simulink model "sampleModel1932"  (R2023a)
settings: Solver=VariableStepAuto  StartTime=0.0  StopTime=10.0  RelTol=1e-3
libraries: hdlsllib x4, simulink x3
settings Model: Creator=user1  LastModifiedBy=user1

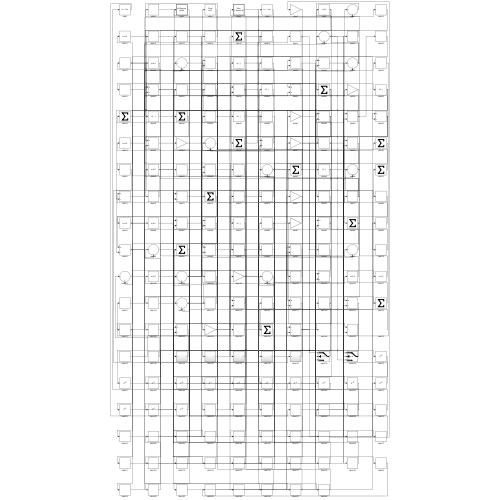
[thumbnail: Simulink's stored preview of the top-level diagram]
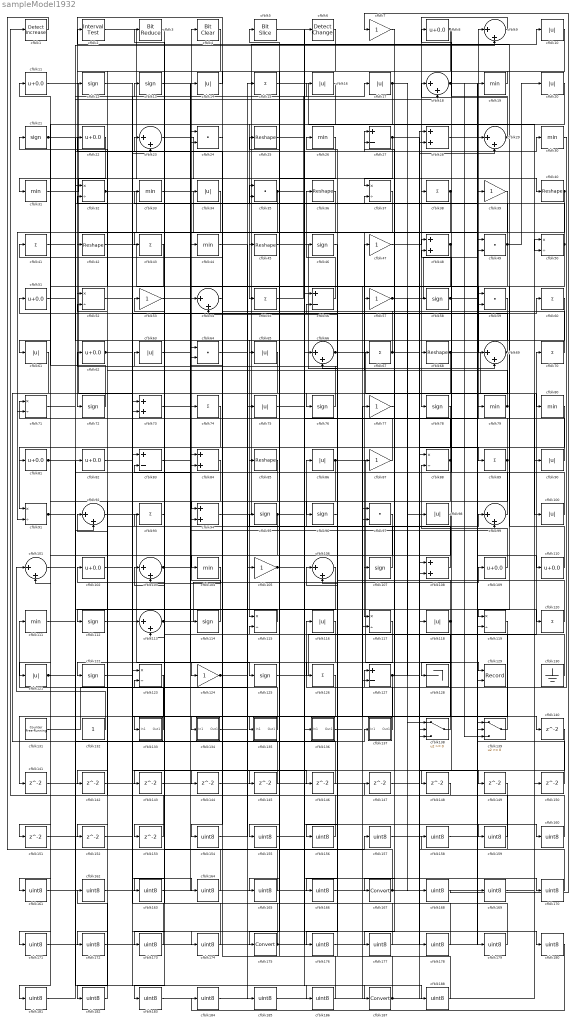
== system sampleModel1932 ==
  cfblk1 : simulink/Logic and Bit Operations/Detect Increase  vinit=0.0  OutDataTypeStr=boolean
      settings: LibrarySourceBlock=|
      | hdlsllib/Logic and Bit
      | Operations/Detect
      | Increase
  cfblk{10,14,16..17,20,34,61,63,65,75,86,90,98,100,116,118,121} (17 alike) : Abs  SaturateOnIntegerOverflow=off
  cfblk{9,18,23,29,54,66,69,92,99,101,103,106,113} (13 alike) : Sum  Inputs=|++
  cfblk{8,11,22,51,62,81..82,102,109..110} (10 alike) : Bias  Bias=0.0  SaturateOnIntegerOverflow=off
  cfblk{19,26,30..31,33,44,79..80,104,111} (10 alike) : MinMax
  cfblk{7,39,47,53,57,77,87,105,124} (9 alike) : Gain
  cfblk{12..13,21,46,58,72,76,78,95..96,107,112,114,122,125} (15 alike) : Signum
  cfblk{28,48,73,84,94,108} (6 alike) : Sum
  cfblk{32,37,50,52,71,88,91,115,117,119,123} (11 alike) : Product  Inputs=*/  RndMeth=Zero  SaturateOnIntegerOverflow=on
  cfblk{15,38,41,43,55,60,67,70,74,89,93,120,126} (13 alike) : Sum  Inputs=+
  cfblk{27,56,83,127} (4 alike) : Sum  Inputs=+-
  cfblk128 : Terminator
  cfblk129 : Record  FileSettingsInternal="{\"entries\":[{\"content\":{\"excelSettings\":{\"content\":{},\"type\":\"Streamout.ExcelSettings\"}},\"type\":\"Streamout.FileSettingStorage\",\"uuid\":\"\"}],\"packageUris\":[\"http:\\/\\/schema.mathworks.com\\/mf0\\/streamout_blocks\\/R2020a\"],\"version\":\"1.0\"}"  Layout=[1 1]  SignalsInternal="{\"entries\":[{\"content\":{\"signals\":[{\"content\":{\"blockPath\":[],\"dimensions\":[1],\"domain\":\"\",\"lineColor\":\"#a2142f\",\"plots\":[1],\"port\":1,\"signalID\":5289,\"signalName\":\"XY Graph:1\"},\"type\":\"RecordBlkView.Signal\",\"uuid\":\"\"},{\"content\":{\"blockPath\":[],\"dimensions\":[1],\"domain\":\"\",\"lineColor\":\"#139fff\",\"plots\":[1],\"port\":2,\"signalID\":5292,\"signalName\":\"XY Graph:2\"},\"type\":\"RecordBlkView.Signal\",\"uuid\":\"\"}]},\"type\":\"RecordBlkView.InputSignals\",\"uuid\":\"\"}],\"packageUris\":[\"http:\\/\\/schema.mathworks.com\\/mf0\\/streamout_blocks\\/R2020a\"],\"version\":\"1.0\"}"  VisualizationBindings="{\"xyplotplugin\":{\"info\":[{\"series\":[{\"bindingParametersList\":[{\"parameter\":\"X-Axis\",\"signalID\":5289,\"signalName\":\"XY Graph:1\"},{\"parameter\":\"Y-Axis\",\"signalID\":5292,\"signalName\":\"XY Graph:2\"}],\"seriesID\":37715}],\"subplotID\":1}]}}"  CompatibilityTag=XY  st=-1
  cfblk130 : Ground
  cfblk131 : hdlsllib/Sources/Counter Free-Running  NumBits=16  tsamp=-1
  cfblk132 : Constant  SampleTime=-1
  cfblk133 : Subsystem
      settings: LibrarySourceBlock=|
      | hdlsllib/Ports &
      | Subsystems/Subsystem
  cfblk134 : Subsystem
      settings: LibrarySourceBlock=|
      | hdlsllib/Ports &
      | Subsystems/Subsystem
  cfblk135 : Subsystem
      settings: LibrarySourceBlock=|
      | hdlsllib/Ports &
      | Subsystems/Subsystem
  cfblk136 : Subsystem
      settings: LibrarySourceBlock=|
      | hdlsllib/Ports &
      | Subsystems/Subsystem
  cfblk137 : Subsystem
      settings: LibrarySourceBlock=|
      | hdlsllib/Ports &
      | Subsystems/Subsystem
  cfblk138 : Switch  SaturateOnIntegerOverflow=off  InputSameDT=off
  cfblk139 : Switch  SaturateOnIntegerOverflow=off  InputSameDT=off
  cfblk{140..153} (14 alike) : Delay  SampleTime=1
  cfblk{154..166,168..174,176..186,188} (32 alike) : DataTypeConversion  OutDataTypeStr=uint8  SaturateOnIntegerOverflow=off  RndMeth=Floor
  cfblk167 : DataTypeConversion  SaturateOnIntegerOverflow=off  RndMeth=Floor
  cfblk175 : DataTypeConversion  SaturateOnIntegerOverflow=off  RndMeth=Floor
  cfblk187 : DataTypeConversion  SaturateOnIntegerOverflow=off  RndMeth=Floor
  cfblk2 : hdlsllib/Logic and Bit Operations/Interval Test  IntervalClosedRight=on  uplimit=0.5  IntervalClosedLeft=on  lowlimit=-0.5  OutDataTypeStr=boolean
  cfblk{24,35,49,59,64,97} (6 alike) : DotProduct  OutDataTypeStr=Inherit: Inherit via internal rule
  cfblk{25,36,40,42,45,68,85} (7 alike) : Reshape
  cfblk3 : hdlsllib/Logic and Bit Operations/Bit Reduce  mode=AND
  cfblk4 : simulink/Logic and Bit Operations/Bit Clear  iBit=0
      settings: LibrarySourceBlock=|
      | hdlsllib/Logic and Bit
      | Operations/Bit Clear
  cfblk5 : hdlsllib/Logic and Bit Operations/Bit Slice  lidx=7  ridx=0
  cfblk6 : simulink/Logic and Bit Operations/Detect Change  vinit=0  OutDataTypeStr=boolean
      settings: LibrarySourceBlock=|
      | hdlsllib/Logic and Bit
      | Operations/Detect
      | Change
  wires:
  cfblk86/1 -> cfblk129/1, cfblk113/2
  cfblk114/1 -> cfblk4/1
  cfblk133/1(Out1) -> cfblk111/1
  cfblk92/1 -> cfblk124/1
  cfblk90/1 -> cfblk9/1
  cfblk78/1 -> cfblk91/1
  cfblk14/1 -> cfblk72/1
  cfblk56/1 -> cfblk36/1
  cfblk55/1 -> cfblk17/1
  cfblk9/1 -> cfblk78/1
  cfblk49/1 -> cfblk25/1, cfblk20/1, cfblk166/1
  cfblk30/1 -> cfblk116/1
  cfblk107/1 -> cfblk21/1
  cfblk113/1 -> cfblk109/1, cfblk125/1
  cfblk137/1(Out1) -> cfblk127/1
  cfblk126/1 -> cfblk133/1(In1)
  cfblk115/1 -> cfblk112/1
  cfblk63/1 -> cfblk60/1
  cfblk37/1 -> cfblk117/1
  cfblk60/1 -> cfblk115/1
  cfblk118/1 -> cfblk54/2, cfblk143/1
  cfblk108/1 -> cfblk86/1
  cfblk35/1 -> cfblk91/2, cfblk160/1
  cfblk94/1 -> cfblk10/1
  cfblk25/1 -> cfblk40/1
  cfblk125/1 -> cfblk70/1
  cfblk130/1 -> cfblk115/2
  cfblk96/1 -> cfblk126/1
  cfblk139/1 -> cfblk95/1
  cfblk21/1 -> cfblk113/1, cfblk65/1
  cfblk110/1 -> cfblk2/1
  cfblk109/1 -> cfblk88/2
  cfblk132/1 -> cfblk101/1
  cfblk106/1 -> cfblk175/1
  cfblk31/1 -> cfblk38/1
  cfblk38/1 -> cfblk128/1, cfblk155/1
  cfblk100/1 -> cfblk53/1
  cfblk32/1 -> cfblk139/2, cfblk179/1
  cfblk4/1 -> cfblk42/1
  cfblk68/1 -> cfblk80/1, cfblk71/2
  cfblk73/1 -> cfblk30/1
  cfblk42/1 -> cfblk69/1
  cfblk70/1 -> cfblk41/1
  cfblk7/1 -> cfblk167/1
  cfblk47/1 -> cfblk48/1
  cfblk61/1 -> cfblk137/1(In1)
  cfblk89/1 -> cfblk107/1, cfblk54/1
  cfblk11/1 -> cfblk87/1
  cfblk117/1 -> cfblk122/1
  cfblk2/1 -> cfblk108/2
  cfblk36/1 -> cfblk135/1(In1)
  cfblk45/1 -> cfblk69/2
  cfblk52/1 -> cfblk39/1
  cfblk16/1 -> cfblk94/1
  cfblk23/1 -> cfblk55/1
  cfblk19/1 -> cfblk12/1
  cfblk20/1 -> cfblk45/1
  cfblk127/1 -> cfblk58/1, cfblk29/2, cfblk27/2, cfblk141/1, cfblk168/1
  cfblk27/1 -> cfblk37/1, cfblk149/1
  cfblk111/1 -> cfblk120/1
  cfblk22/1 -> cfblk31/1
  cfblk69/1 -> cfblk73/2, cfblk51/1
  cfblk10/1 -> cfblk52/1
  cfblk40/1 -> cfblk81/1, cfblk67/1
  cfblk102/1 -> cfblk24/1
  cfblk51/1 -> cfblk29/1
  cfblk120/1 -> cfblk63/1
  cfblk103/1 -> cfblk14/1, cfblk99/2, cfblk37/2
  cfblk18/1 -> cfblk139/1, cfblk139/3
  cfblk57/1 -> cfblk19/1, cfblk138/1
  cfblk91/1 -> cfblk84/1, cfblk186/1
  cfblk76/1 -> cfblk62/1
  cfblk50/1 -> cfblk3/1, cfblk129/2, cfblk119/1, cfblk84/2
  cfblk121/1 -> cfblk13/1, cfblk181/1
  cfblk53/1 -> cfblk24/2
  cfblk24/1 -> cfblk104/1
  cfblk8/1 -> cfblk68/1, cfblk85/1
  cfblk124/1 -> cfblk105/1, cfblk138/2
  cfblk99/1 -> cfblk48/2
  cfblk48/1 -> cfblk117/2, cfblk145/1
  cfblk65/1 -> cfblk134/1(In1)
  cfblk136/1(Out1) -> cfblk77/1
  cfblk46/1 -> cfblk76/1
  cfblk15/1 -> cfblk50/2
  cfblk134/1(Out1) -> cfblk99/1
  cfblk95/1 -> cfblk151/1, cfblk170/1
  cfblk34/1 -> cfblk121/1
  cfblk138/1 -> cfblk102/1
  cfblk13/1 -> cfblk114/1
  cfblk62/1 -> cfblk56/2, cfblk16/1
  cfblk39/1 -> cfblk43/1
  cfblk29/1 -> cfblk8/1, cfblk18/1
  cfblk41/1 -> cfblk35/1
  cfblk79/1 -> cfblk47/1, cfblk52/2
  cfblk87/1 -> cfblk71/1
  cfblk75/1 -> cfblk136/1(In1)
  cfblk43/1 -> cfblk101/2
  cfblk88/1 -> cfblk57/1, cfblk96/1
  cfblk135/1(Out1) -> cfblk23/1
  cfblk105/1 -> cfblk46/1, cfblk79/1
  cfblk104/1 -> cfblk103/2
  cfblk131/1 -> cfblk15/1
  cfblk71/1 -> cfblk9/2
  cfblk81/1 -> cfblk92/2, cfblk18/2
  cfblk72/1 -> cfblk11/1
  cfblk17/1 -> cfblk61/1, cfblk98/1
  cfblk5/1 -> cfblk187/1
  cfblk101/1 -> cfblk27/1
  cfblk80/1 -> cfblk94/2
  cfblk67/1 -> cfblk22/1, cfblk89/1
  cfblk58/1 -> cfblk110/1, cfblk148/1
  cfblk66/1 -> cfblk100/1, cfblk138/3
  cfblk83/1 -> cfblk35/2
  cfblk64/1 -> cfblk140/1
  cfblk141/1 -> cfblk56/1
  cfblk84/1 -> cfblk142/1
  cfblk142/1 -> cfblk92/1
  cfblk143/1 -> cfblk88/1
  cfblk54/1 -> cfblk144/1
  cfblk144/1 -> cfblk127/2
  cfblk145/1 -> cfblk32/1
  cfblk122/1 -> cfblk146/1
  cfblk146/1 -> cfblk103/1
  cfblk148/1 -> cfblk1/1
  cfblk150/1 -> cfblk49/1
  cfblk151/1 -> cfblk23/2
  cfblk119/1 -> cfblk152/1
  cfblk116/1 -> cfblk153/1
  cfblk153/1 -> cfblk73/1
  cfblk6/1 -> cfblk154/1
  cfblk154/1 -> cfblk75/1
  cfblk155/1 -> cfblk6/1
  cfblk59/1 -> cfblk156/1
  cfblk156/1 -> cfblk32/2
  cfblk1/1 -> cfblk157/1
  cfblk157/1 -> cfblk59/1
  cfblk149/1 -> cfblk158/1
  cfblk158/1 -> cfblk59/2
  cfblk147/1 -> cfblk159/1
  cfblk159/1 -> cfblk108/1
  cfblk160/1 -> cfblk147/1
  cfblk74/1 -> cfblk161/1
  cfblk161/1 -> cfblk50/1
  cfblk162/1 -> cfblk74/1
  cfblk93/1 -> cfblk163/1
  cfblk163/1 -> cfblk64/1
  cfblk12/1 -> cfblk164/1
  cfblk164/1 -> cfblk93/1
  cfblk26/1 -> cfblk165/1
  cfblk165/1 -> cfblk64/2
  cfblk166/1 -> cfblk26/1
  cfblk167/1 -> cfblk119/2, cfblk83/2
  cfblk168/1 -> cfblk7/1
  cfblk28/1 -> cfblk169/1
  cfblk169/1 -> cfblk150/1
  cfblk170/1 -> cfblk28/1
  cfblk85/1 -> cfblk171/1
  cfblk171/1 -> cfblk28/2
  cfblk123/1 -> cfblk172/1
  cfblk172/1 -> cfblk49/2
  cfblk3/1 -> cfblk173/1
  cfblk173/1 -> cfblk123/1
  cfblk152/1 -> cfblk174/1
  cfblk174/1 -> cfblk123/2
  cfblk175/1 -> cfblk66/1, cfblk83/1
  cfblk98/1 -> cfblk176/1
  cfblk176/1 -> cfblk106/1
  cfblk77/1 -> cfblk177/1
  cfblk177/1 -> cfblk106/2
  cfblk33/1 -> cfblk178/1
  cfblk178/1 -> cfblk34/1
  cfblk179/1 -> cfblk33/1
  cfblk82/1 -> cfblk180/1
  cfblk181/1 -> cfblk82/1
  cfblk97/1 -> cfblk182/1
  cfblk182/1 -> cfblk162/1
  cfblk140/1 -> cfblk183/1
  cfblk183/1 -> cfblk97/1
  cfblk180/1 -> cfblk184/1
  cfblk184/1 -> cfblk97/2
  cfblk44/1 -> cfblk185/1
  cfblk185/1 -> cfblk118/1
  cfblk186/1 -> cfblk44/1
  cfblk187/1 -> cfblk66/2, cfblk90/1
  cfblk112/1 -> cfblk188/1
  cfblk188/1 -> cfblk5/1

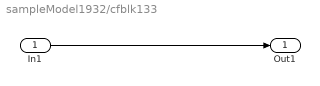
== system sampleModel1932/cfblk133 ==
  In1 : Inport
  Out1 : Outport
  wires:
  In1/1 -> Out1/1

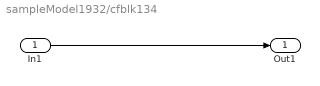
== system sampleModel1932/cfblk134 ==
  In1 : Inport
  Out1 : Outport
  wires:
  In1/1 -> Out1/1

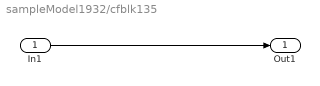
== system sampleModel1932/cfblk135 ==
  In1 : Inport
  Out1 : Outport
  wires:
  In1/1 -> Out1/1

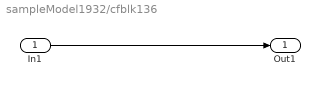
== system sampleModel1932/cfblk136 ==
  In1 : Inport
  Out1 : Outport
  wires:
  In1/1 -> Out1/1

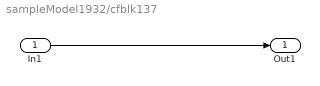
== system sampleModel1932/cfblk137 ==
  In1 : Inport
  Out1 : Outport
  wires:
  In1/1 -> Out1/1
